simulink model "batteryCharger"  (R2021a)
settings: Solver=VariableStepAuto  StartTime=0.0  StopTime=0.05  RelTol=1e-3
libraries: spsSeriesRLCBranchLib x2, spsCurrentMeasurementLib x2, spsVoltageMeasurementLib x2, spsSeriesRLCLoadLib x1, spsDCVoltageSourceLib x1, spsDiodeLib x1, spsMosfetLib x1, spspowerguiLib x1
settings Model: Creator=ishit  LastModifiedBy=user
settings SolverCC: AlgebraicLoopSolver=TrustRegion
settings DebuggingCC: SFMachineParentedDataDiag=warning

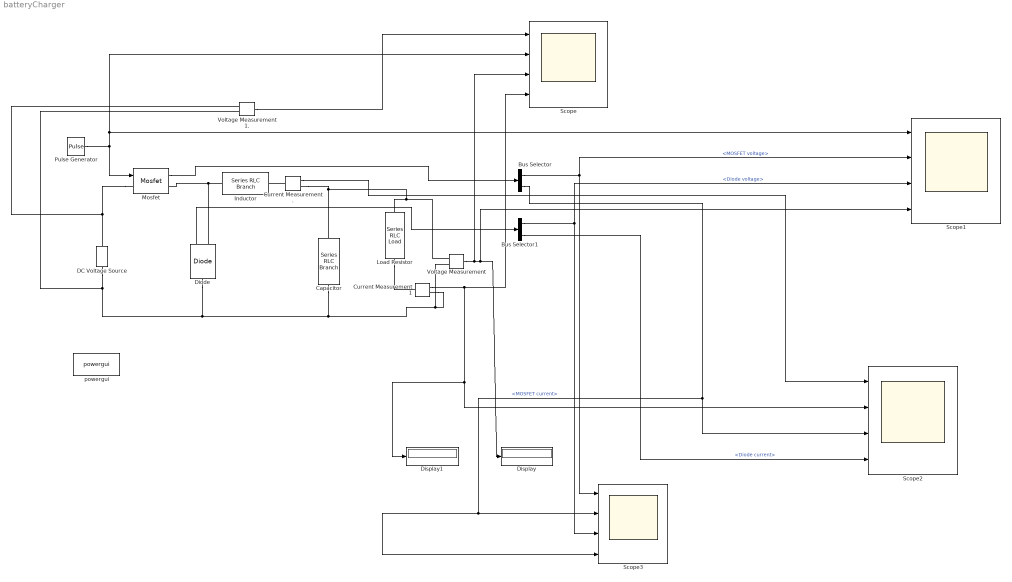
== system batteryCharger ==
  " Load Resistor" : spsSeriesRLCLoadLib/Series RLC Load  LConnTagsString=a  RConnTagsString=__new0  NominalVoltage=48  NominalFrequency=50e3  ActivePower=96  InductivePower=0  CapacitivePower=0  Setx0=off  InitialVoltage=0  SetiL0=off  InitialCurrent=0  Measurements=None  LoadType=constant Z
  Bus Selector : BusSelector  OutputSignals=MOSFET voltage,MOSFET current
  Bus Selector1 : BusSelector  OutputSignals=Diode voltage,Diode current
  Capacitor : spsSeriesRLCBranchLib/Series RLC Branch  LConnTagsString=__new0  RConnTagsString=__new0  BranchType=C  Resistance=1  Inductance=1e-3  SetiL0=off  InitialCurrent=0  Capacitance=4.17e-4  Setx0=off  InitialVoltage=0  Measurements=None
  Current Measurement 1 : spsCurrentMeasurementLib/Current Measurement  PhasorSimulation=off  OutputType=Complex  PSBequivalent=0
  Current Measurement. : spsCurrentMeasurementLib/Current Measurement  PhasorSimulation=off  OutputType=Complex  PSBequivalent=0
  DC Voltage Source : spsDCVoltageSourceLib/DC Voltage Source  Amplitude=48  Measurements=None
  "Diode " : spsDiodeLib/Diode  Ron=0.0005  Lon=0  Vf=0.01  IC=0  UseSnubber=0  Rs=500  Cs=250e-9  Measurements=on
  Display : Display
  Display1 : Display
  Inductor : spsSeriesRLCBranchLib/Series RLC Branch  LConnTagsString=__new0  RConnTagsString=__new0  BranchType=L  Resistance=1  Inductance=3e-4  SetiL0=off  InitialCurrent=0  Capacitance=1e-6  Setx0=off  InitialVoltage=0  Measurements=None
  "Mosfet " : spsMosfetLib/Mosfet  Ron=0.0005  Lon=0  Rd=0.01  Vfd=0  IC=0  Rs=1e5  Cs=inf  Measurements=on
  "Pulse Generator " : DiscretePulseGenerator  PulseType=Time based  Amplitude=5  Period=1/50000  PulseWidth=50
  Scope{,1..3} (4 alike) : Scope  NumInputPorts=4
  "Voltage Measurement " : spsVoltageMeasurementLib/Voltage Measurement  PhasorSimulation=off  OutputType=Complex  PSBequivalent=0
  Voltage Measurement1. : spsVoltageMeasurementLib/Voltage Measurement  PhasorSimulation=off  OutputType=Complex  PSBequivalent=0
  powergui : spspowerguiLib/powergui  Priority=1  SimulationMode=Continuous  SampleTime=50e-6  frequency=60  Iterations=50  frequencyindice=0  Pbase=100e6  ErrMax=1e-4  UnitsV=kV  UnitsW=MW  buscounter=0  FunctionMessages=off  echomessages=off  EnableUseOfTLC=off  CurrentSourceSwitches=off  DisableSnubberDevices=off  DisableRonSwitches=off  DisableVfSwitches=off  DisplayEquations=off  AutomaticDiscreteSolvers=off  SolverType=Tustin/Backward Euler (TBE)  Interpol=off  ExternalGateDelay=off  methode=off  Ts=100  x0status=blocks  SPID=on  SwTol=0  HookPort=off  NonlinearTolerance=1e-4  nMaxIteration=100  ContinueOnMaxIteration=off  RestoreLinks=warning  ResistiveCurrentMeasurement=off  Frange=[0:2:500]  Ylog=off  Xlog=on  ShowGrid=off  save=off  variable=ZData  structure=0  ZoomFFT=off  StartTime=0.0  cycles=1  DisplayStyle=1  fundamental=60  FreqAxis=off  MaxFrequency=1000  frequencyindicesteady=1  RmsSteady=1  display=off
  wires:
  Bus Selector/2 -> Scope3/4, Scope3/2, Scope2/3  "<MOSFET current>"
  Current Measurement 1/1 -> Scope2/2, Display1/1, Scope/4
  "Voltage Measurement "/1 -> Scope/3, Display/1, Scope1/4
  "Mosfet "/1 -> Bus Selector/1
  Voltage Measurement1./1 -> Scope/1
  Bus Selector1/2 -> Scope2/4  "<Diode current>"
  "Diode "/1 -> Bus Selector1/1
  Current Measurement./1 -> Scope2/1
  Bus Selector1/1 -> Scope3/3, Scope1/3  "<Diode voltage>"
  "Pulse Generator "/1 -> Scope1/1, Scope/2, "Mosfet "/1
  Bus Selector/1 -> Scope3/1, Scope1/2  "<MOSFET voltage>"
  connections:
  Capacitor/RConn1 -- Current Measurement 1/RConn1 -- "Voltage Measurement "/LConn2 -- "Diode "/LConn1 -- DC Voltage Source/LConn1 -- Voltage Measurement1./LConn2
  "Mosfet "/RConn1 -- Inductor/LConn1 -- "Diode "/RConn1
  Current Measurement./RConn1 -- Capacitor/LConn1 -- " Load Resistor"/LConn1 -- "Voltage Measurement "/LConn1
  "Mosfet "/LConn1 -- DC Voltage Source/RConn1 -- Voltage Measurement1./LConn1
  Current Measurement./LConn1 -- Inductor/RConn1
  " Load Resistor"/RConn1 -- Current Measurement 1/LConn1
